simulink model "speed_PI_controller_case2"  (R2025b)
settings: Solver=FixedStepAuto  StartTime=0.0  StopTime=7  FixedStep=0.0001  MaxStep=0.0000001  RelTol=1e-3
libraries: slpidlib x1
settings Model: Creator=danfa  LastModifiedBy=danfa

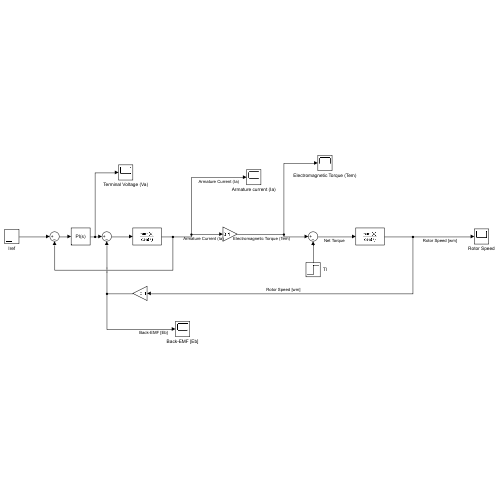
[thumbnail: Simulink's stored preview of the top-level diagram]
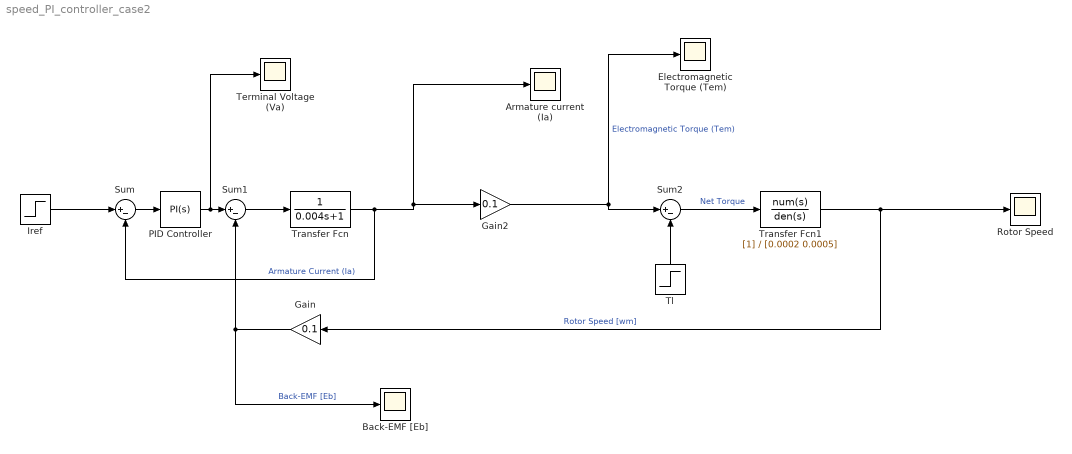
== system speed_PI_controller_case2 ==
  Armature current (Ia) : Scope
      settings: ActiveDisplayYMinimum=-0.180287760691444  ActiveDisplayYMaximum=1.6225898462229962
  Back-EMF [Eb] : Scope
      settings: ActiveDisplayYMinimum=-2.4999991713322394  ActiveDisplayYMaximum=22.49999254199016  DataLoggingVariableName=ScopeData3
  Electromagnetic Torque (Tem) : Scope
      settings: ActiveDisplayYMinimum=-0.01489817903047096  ActiveDisplayYMaximum=0.13408361127423868  DataLoggingVariableName=ScopeData2
  Gain : Gain  Gain=0.1
  Gain2 : Gain  Gain=0.1
  Iref : Step  SampleTime=0
  PID Controller : slpidlib/PID Controller  Controller=PI  Form=Parallel  TimeDomain=Continuous-time  UseExternalTs=off  SampleTime=-1  IntegratorMethod=Forward Euler  FilterMethod=Forward Euler  ControllerParametersSource=internal  P=4.9414  I=6295.1517  UseKiTs=off  D=0  UseExternalDerivativeSource=off  N=100  UseFilter=on  TunerSelectOption=Transfer Function Based (PID Tuner App)  InitialConditionSource=internal  InitialConditionForIntegrator=0  InitialConditionForFilter=0  DifferentiatorICPrevScaledInput=0  ExternalReset=none  TrackingMode=off  Kt=1  LimitOutput=off  SatLimitsSource=internal  UpperSaturationLimit=inf  LowerSaturationLimit=-inf  LinearizeAsGain=on  AntiWindupMode=none  Kb=1  LimitIntegrator=off  UpperIntegratorSaturationLimit=inf  LowerIntegratorSaturationLimit=-inf  POutMin=[]  POutMax=[]  IOutMin=[]  IOutMax=[]  DOutMin=[]  DOutMax=[]  NOutMin=[]  NOutMax=[]  SumOutMin=[]  SumOutMax=[]  SaturationOutMin=[]  SaturationOutMax=[]  PParamMin=[]  PParamMax=[]  IParamMin=[]  IParamMax=[]  DParamMin=[]  DParamMax=[]  NParamMin=[]  NParamMax=[]  KbParamMin=[]  KbParamMax=[]  KtParamMin=[]  KtParamMax=[]  KbOutMin=[]  KbOutMax=[]  KtOutMin=[]  KtOutMax=[]  IntegratorOutMin=[]  IntegratorOutMax=[]  FilterOutMin=[]  FilterOutMax=[]  SumI1OutMin=[]  SumI1OutMax=[]  SumI2OutMin=[]  SumI2OutMax=[]  SumI3OutMin=[]  SumI3OutMax=[]  SumI4OutMin=[]  SumI4OutMax=[]  SumDOutMin=[]  SumDOutMax=[]  DifferentiatorOutMin=[]  DifferentiatorOutMax=[]  FilterDiffOutCoefMin=[]  FilterDiffOutCoefMax=[]  ReciprocalOutMin=[]  ReciprocalOutMax=[]  SumDenOutMin=[]  SumDenOutMax=[]  SumNumOutMin=[]  SumNumOutMax=[]  DivideOutMin=[]  DivideOutMax=[]  UdiffTsProdOutMin=[]  UdiffTsProdOutMax=[]  NTsProdOutMin=[]  NTsProdOutMax=[]  UintegralTsProdOutMin=[]  UintegralTsProdOutMax=[]  UngainTsProdOutMin=[]  UngainTsProdOutMax=[]  ClampingZeroOutDataTypeStr=Inherit: Inherit via back propagation  ClampingZeroOutMin=[]  ClampingZeroOutMax=[]  FilterDenConstantOutDataTypeStr=Inherit: Inherit via back propagation  FilterDenConstantOutMin=[]  FilterDenConstantOutMax=[]  PCopyOutDataTypeStr=Inherit: Inherit via back propagation  PCopyOutMin=[]  PCopyOutMax=[]  NCopyOutDataTypeStr=Inherit: Inherit via back propagation  NCopyOutMin=[]  NCopyOutMax=[]  IntegratorContinuousStateAttributes=''  IntegratorStateMustResolveToSignalObject=off  IntegratorRTWStateStorageClass=Auto  FilterContinuousStateAttributes=''  FilterStateMustResolveToSignalObject=off  FilterRTWStateStorageClass=Auto  ParallelPVariant=InternalParameters  IdealPVariant=Disabled  IVariant=InternalParameters  DVariant=Disabled  IntegratorVariant=Continuous  SatVariant=Disabled  AWVariant=Passthrough  PCopyVariant=Disabled  TRVariant=Disabled  FdbkBlocksVariant=Forward  IdealPFdbkVariant=Disabled  SatFdbkVariant=Disabled  DerivativeFilterVariant=Disabled  NVariant=Disabled  NCopyVariant=Disabled_SignalSpec  FilterICVariant=Disabled  IntegratorICVariant=InternalICs  ExternalResetVariant=Disabled  TRSumVariant=Passthrough  SumFdbkVariant=Disabled  SumVariant=Sum_PI  TsampFilterVariant=InternalTs  TsampNgainVariant=Passthrough  TsampIntegralVariant=Disabled_SignalSpec  ExternalSaturationOutDataTypeStr=Inherit: Same as second input  DerivativeSourceVariant=Disabled  PreIntVariant=InternalPreInt
  Rotor Speed : Scope
      settings: ActiveDisplayYMinimum=-24.999991713322391  ActiveDisplayYMaximum=224.99992541990159
  Sum : Sum  Inputs=|+-
  Sum1 : Sum  Inputs=|+-
  Sum2 : Sum  Inputs=|+-
  Terminal Voltage (Va) : Scope
      settings: ActiveDisplayYMinimum=-5.6920889854492351  ActiveDisplayYMaximum=23.933633623075536  DataLoggingVariableName=ScopeData4
  Tl : Step  Time=7  After=0.05  SampleTime=0
  Transfer Fcn : TransferFcn  Denominator=[0.004 1]
  Transfer Fcn1 : TransferFcn  Denominator=[0.0002 0.0005]
  wires:
  Iref/1 -> Sum/1
  Transfer Fcn/1 -> Sum/2, Armature current (Ia)/1, Gain2/1  "Armature Current (Ia)"
  Sum/1 -> PID Controller/1
  Gain2/1 -> Sum2/1, Electromagnetic Torque (Tem)/1  "Electromagnetic Torque (Tem)"
  Sum2/1 -> Transfer Fcn1/1  "Net Torque"
  Tl/1 -> Sum2/2
  Transfer Fcn1/1 -> Rotor Speed/1, Gain/1  "Rotor Speed [wm]"
  Gain/1 -> Sum1/2, Back-EMF [Eb]/1  "Back-EMF [Eb]"
  PID Controller/1 -> Terminal Voltage (Va)/1, Sum1/1
  Sum1/1 -> Transfer Fcn/1
